simulink library "INT_CoPT_TrqDesCoord"  (R2016b)
settings: Solver=VariableStepAuto  StartTime=0.0  StopTime=10.0  RelTol=1e-3
settings Model: Creator=Administrator  LastModifiedBy=Administrator

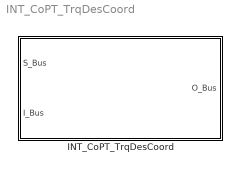
== system INT_CoPT_TrqDesCoord ==
  INT_CoPT_TrqDesCoord : Subsystem

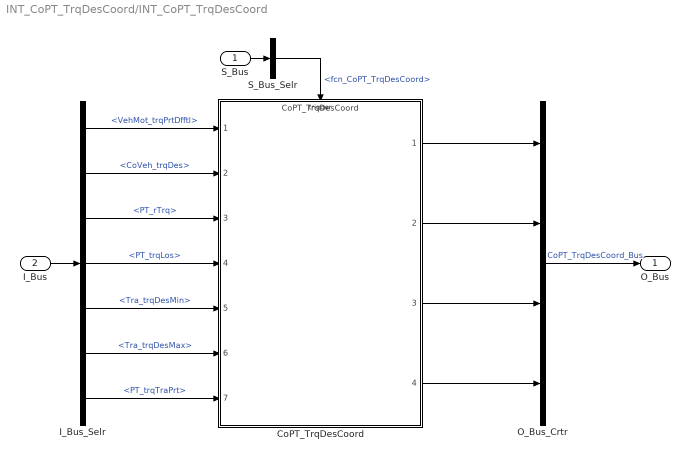
== system INT_CoPT_TrqDesCoord/INT_CoPT_TrqDesCoord ==
  S_Bus : Inport
  I_Bus : Inport  Port=2
  CoPT_TrqDesCoord : ModelReference  ModelNameDialog=CoPT_TrqDesCoord  SimulationMode=Normal  ModelReferenceVersion=1.5  TriggerPortName=function  TriggerPortTriggerType=function-call  TriggerPortStatesWhenEnabling=held
  I_Bus_Selr : BusSelector  OutputSignals=VehMot_trqPrtDfftl,CoVeh_trqDes,PT_rTrq,PT_trqLos,Tra_trqDesMin,Tra_trqDesMax,PT_trqTraPrt
  O_Bus_Crtr : BusCreator  Inputs=4
  S_Bus_Selr : BusSelector  OutputSignals=fcn_CoPT_TrqDesCoord
  O_Bus : Outport
  wires:
  S_Bus_Selr/1 -> CoPT_TrqDesCoord/Trigger  "<fcn_CoPT_TrqDesCoord>"
  S_Bus/1 -> S_Bus_Selr/1
  I_Bus/1 -> I_Bus_Selr/1
  I_Bus_Selr/1 -> CoPT_TrqDesCoord/1  "<VehMot_trqPrtDfftl>"
  I_Bus_Selr/2 -> CoPT_TrqDesCoord/2  "<CoVeh_trqDes>"
  I_Bus_Selr/3 -> CoPT_TrqDesCoord/3  "<PT_rTrq>"
  I_Bus_Selr/4 -> CoPT_TrqDesCoord/4  "<PT_trqLos>"
  I_Bus_Selr/5 -> CoPT_TrqDesCoord/5  "<Tra_trqDesMin>"
  I_Bus_Selr/6 -> CoPT_TrqDesCoord/6  "<Tra_trqDesMax>"
  I_Bus_Selr/7 -> CoPT_TrqDesCoord/7  "<PT_trqTraPrt>"
  O_Bus_Crtr/1 -> O_Bus/1  "CoPT_TrqDesCoord_Bus"
  CoPT_TrqDesCoord/1 -> O_Bus_Crtr/1
  CoPT_TrqDesCoord/2 -> O_Bus_Crtr/2
  CoPT_TrqDesCoord/3 -> O_Bus_Crtr/3
  CoPT_TrqDesCoord/4 -> O_Bus_Crtr/4
